simulink model "quadcopter_process_test"  (R2015b)
settings: Solver=VariableStepAuto  StartTime=0.0  StopTime=2  RelTol=1e-3
undefined symbols (not defined in the file): h
libraries: vrlib x2
settings Model: Creator=Daniel  LastModifiedBy=mgreiff

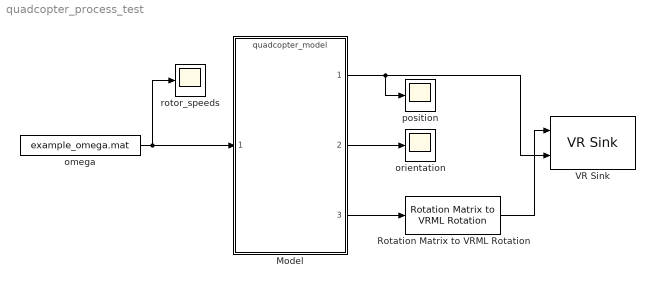
== system quadcopter_process_test ==
  Model : ModelReference  ModelNameDialog=quadcopter_model.mdl  SimulationMode=Normal  ModelReferenceVersion=1.114  CopyOfModelName=quadcopter_model.mdl
  Rotation Matrix to VRML Rotation : vrlib/Utilities/Rotation Matrix to VRML Rotation  maxzero=1e-12
  VR Sink : vrlib/VR Sink  InstantiateOnLoad=on  SampleTime=0.1  ViewEnable=on  RemoteChange=off  RemoteView=off  FieldsWritten=copter.rotation.4.1.1.double#copter.translation.3.1.1.double  WorldFileName=copter_world.wrl  AutoView=on  VideoDimensions=[]  AllowVariableSize=off
  omega : FromFile  FileName=example_omega.mat  SampleTime=h
  orientation : Scope
  position : Scope
  rotor_speeds : Scope
  wires:
  omega/1 -> rotor_speeds/1, Model/1
  Rotation Matrix to VRML Rotation/1 -> VR Sink/1
  Model/2 -> orientation/1
  Model/3 -> Rotation Matrix to VRML Rotation/1
  Model/1 -> position/1, VR Sink/2
